simulink model "module_8_exercise_1"  (R2022a)
settings: Solver=ode4  StartTime=0.0  StopTime=10.0  FixedStep=0.1  RelTol=1e-3
settings Model: Creator=hntran  LastModifiedBy=hntran

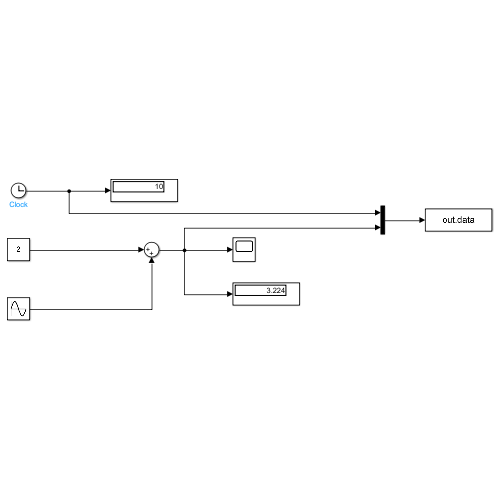
[thumbnail: Simulink's stored preview of the top-level diagram]
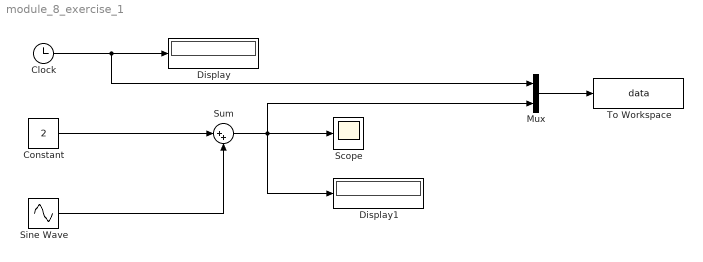
== system module_8_exercise_1 ==
  Clock : Clock
  Constant : Constant  Value=2
  Display : Display
  Display1 : Display
  Mux : Mux  Inputs=2
  Scope : Scope
  Sine Wave : Sin  Amplitude=3  Frequency=2  Phase=pi/2  SampleTime=0
  Sum : Sum  Inputs=|++
  To Workspace : ToWorkspace  VariableName=data  SampleTime=-1
  wires:
  Sine Wave/1 -> Sum/2
  Constant/1 -> Sum/1
  Clock/1 -> Mux/1, Display/1
  Sum/1 -> Mux/2, Display1/1, Scope/1
  Mux/1 -> To Workspace/1
